simulink model "cam1"  (R2016b)
settings: Solver=ode3  StartTime=0.0  StopTime=1000.0  FixedStep=0.2  RelTol=1e-3  EnableMultiTasking=on
undefined symbols (not defined in the file or in its folder): Angular, Linear
libraries: robotlib x3, simulink x3, realtime_pacer_lib x2
settings Model: Creator=esther  LastModifiedBy=esther
settings DataIOCC: SaveFormat=Array
settings OptimizationCC: MaxStackSize=64
settings DebuggingCC: ParameterTunabilityLossMsg=error
settings HardwareCC: ProdBitPerPointer=32  ProdBitPerSizeT=32  ProdBitPerPtrDiffT=32  ProdLargestAtomicFloat=None  ProdIntDivRoundTo=Undefined  ProdEndianess=Unspecified  ProdWordSize=32  ProdHWDeviceType=Generic->Unspecified (assume 32-bit Generic)
settings RTWCC: SystemTargetFile=ert.tlc  HardwareBoard=Robot Operating System (ROS)  TLCOptions="-aInlineSetEventsForThisBaseRateFcn=TLC_FALSE -aSuppressMultiTaskScheduler=TLC_FALSE  -aRateBasedStepFcn=0"  TemplateMakefile=ert_default_tmf  Description=Embedded Coder  GenerateReport=on  RTWVerbose=off  Toolchain=Catkin  IncludeHyperlinkInReport=on  LaunchReport=on  TargetLang=C++  GenerateTraceInfo=on  GenerateTraceReport=on  GenerateTraceReportSl=on  GenerateTraceReportSf=on  GenerateTraceReportEml=on
settings CodeAppCC: ForceParamTrailComments=on  OperatorAnnotations=on  SimulinkDataObjDesc=on  SFDataObjDesc=on  MATLABFcnDesc=on  InsertBlockDesc=on  MATLABSourceComments=on
settings ERTTargetCC: MultiInstanceERTCode=on  CodeInterfacePackaging=C++ class  SupportContinuousTime=on  SupportVariableSizeSignals=on  RootIOFormat=Structure reference

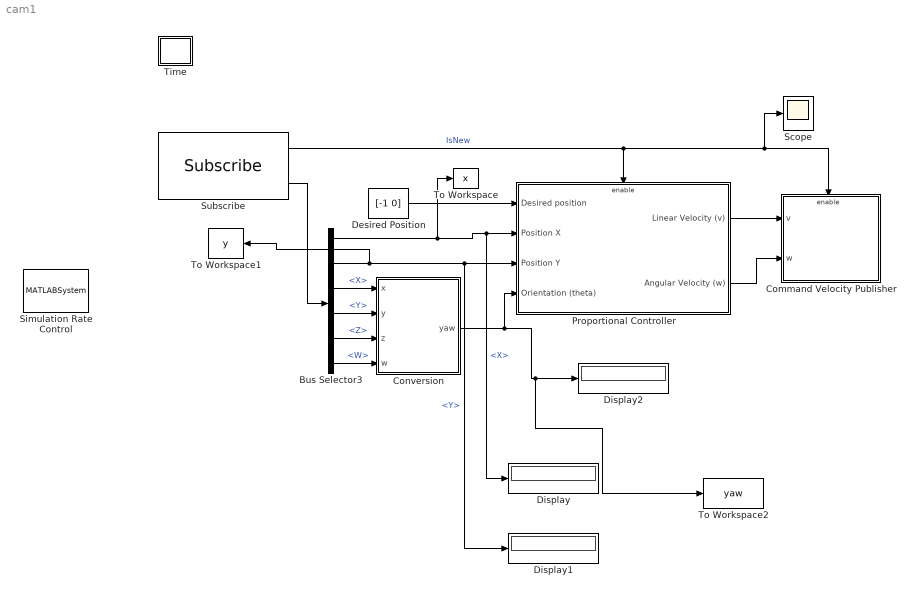
== system cam1 ==
  Bus Selector3 : BusSelector  OutputSignals=Pose.Pose.Position.X,Pose.Pose.Position.Y,Pose.Pose.Orientation.X,Pose.Pose.Orientation.Y,Pose.Pose.Orientation.Z,Pose.Pose.Orientation.W
  Command Velocity Publisher : Subsystem
  Conversion : MATLAB Function  TreatAsAtomicUnit=on
  Desired Position : Constant  Value=[-1 0]  SampleTime=-1
  Display : Display
  Display1 : Display
  Display2 : Display
  Proportional Controller : Subsystem
  Scope : Scope
  Simulation Rate Control : MATLABSystem  System=ExampleHelperSimulationRateControl  SampleTime=0.02
      mask Type: ExampleHelperSimulationRateControl
      mask Display: disp('Rate Control');
  Subscribe : robotlib/Subscribe  SourceLibraryInfo=This block requires Robotics System Toolbox  topicSource=Select from ROS network  topic=/robot_0/pose  messageType=nav_msgs/Odometry  sampleTime=-1  messageQueueLength=51
  Time : Subsystem
  To Workspace : ToWorkspace  VariableName=x  SampleTime=-1
  To Workspace1 : ToWorkspace  VariableName=y  SampleTime=-1
  To Workspace2 : ToWorkspace  VariableName=yaw  SampleTime=-1
  wires:
  Subscribe/2 -> Bus Selector3/1
  Desired Position/1 -> Proportional Controller/1(Desired position)
  Proportional Controller/1(Linear Velocity (v)) -> Command Velocity Publisher/1(v)
  Subscribe/1 -> Command Velocity Publisher/Enable, Scope/1, Proportional Controller/Enable  "IsNew"
  Bus Selector3/3 -> Conversion/1(x)  "<X>"
  Bus Selector3/4 -> Conversion/2(y)  "<Y>"
  Bus Selector3/5 -> Conversion/3(z)  "<Z>"
  Bus Selector3/6 -> Conversion/4(w)  "<W>"
  Conversion/1(yaw) -> Proportional Controller/4(Orientation (theta)), To Workspace2/1, Display2/1
  Bus Selector3/2 -> To Workspace1/1, Display1/1, Proportional Controller/3(Position Y)  "<Y>"
  Proportional Controller/2(Angular Velocity (w)) -> Command Velocity Publisher/2(w)
  Bus Selector3/1 -> To Workspace/1, Display/1, Proportional Controller/2(Position X)  "<X>"

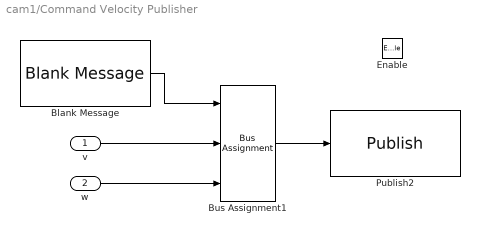
== system cam1/Command Velocity Publisher ==
  v : Inport
  w : Inport  Port=2
  Enable : EnablePort
  Blank Message : robotlib/Blank Message  SourceLibraryInfo=This block requires Robotics System Toolbox  messageType=geometry_msgs/Twist  SampleTime=inf
  Bus Assignment1 : BusAssignment  DialogController=Simulink.DDGSource_BusAssignment  AssignedSignals=Linear.X,Angular.Z
  Publish2 : robotlib/Publish  SourceLibraryInfo=This block requires Robotics System Toolbox  topicSource=Select from ROS network  topic=/robot_0/cmd_vel  messageType=geometry_msgs/Twist  messageQueueLength=105
  wires:
  Bus Assignment1/1 -> Publish2/1
  Blank Message/1 -> Bus Assignment1/1
  v/1 -> Bus Assignment1/2
  w/1 -> Bus Assignment1/3

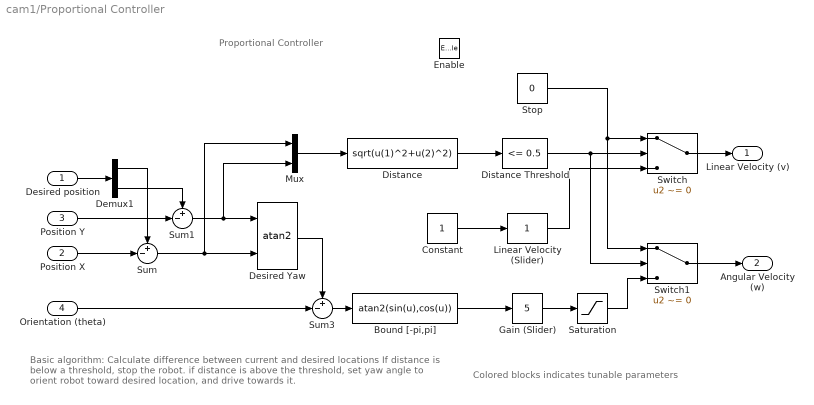
== system cam1/Proportional Controller ==
  note: Proportional Controller
  note: Basic algorithm:
      | Calculate difference between current and desired locations
      | If distance is below a threshold, stop the robot.
      | if distance is above the threshold, set yaw angle to orient robot toward desired location, and drive towards it.
  note: Colored blocks indicates tunable parameters
  Desired position : Inport
  Position X : Inport  Port=2
  Position Y : Inport  Port=3
  Orientation (theta) : Inport  Port=4
  Enable : EnablePort
  Bound [-pi,pi] : Fcn  Expr=atan2(sin(u),cos(u))
  Constant : Constant
  Demux1 : Demux  Outputs=2
  Desired Yaw : Trigonometry  Operator=atan2
  Distance : Fcn  Expr=sqrt(u(1)^2+u(2)^2)
  Distance Threshold : simulink/Logic and Bit Operations/Compare To Constant  relop=<=  const=0.5  OutDataTypeStr=boolean
  Gain (Slider) : simulink/Math Operations/Slider Gain  low=1  gain=5  high=10
  Linear Velocity (Slider) : simulink/Math Operations/Slider Gain  low=0  gain=1  high=2
  Mux : Mux  Inputs=2
  Saturation : Saturate
  Stop : Constant  Value=0
  Sum : Sum  Inputs=+-|
  Sum1 : Sum  Inputs=+-|
  Sum3 : Sum  Inputs=+-|
  Switch : Switch  Criteria=u2 ~= 0
  Switch1 : Switch  Criteria=u2 ~= 0
  Linear Velocity (v) : Outport
  Angular Velocity (w) : Outport  Port=2
  wires:
  Demux1/1 -> Sum/1
  Demux1/2 -> Sum1/1
  Sum1/1 -> Desired Yaw/1, Mux/2
  Constant/1 -> Linear Velocity (Slider)/1
  Desired position/1 -> Demux1/1
  Position Y/1 -> Sum1/2
  Position X/1 -> Sum/2
  Distance/1 -> Distance Threshold/1
  Mux/1 -> Distance/1
  Bound [-pi,pi]/1 -> Gain (Slider)/1
  Orientation (theta)/1 -> Sum3/2
  Desired Yaw/1 -> Sum3/1
  Sum/1 -> Desired Yaw/2, Mux/1
  Distance Threshold/1 -> Switch/2, Switch1/2
  Gain (Slider)/1 -> Saturation/1
  Saturation/1 -> Switch1/3
  Stop/1 -> Switch/1, Switch1/1
  Sum3/1 -> Bound [-pi,pi]/1
  Switch/1 -> Linear Velocity (v)/1
  Linear Velocity (Slider)/1 -> Switch/3
  Switch1/1 -> Angular Velocity (w)/1

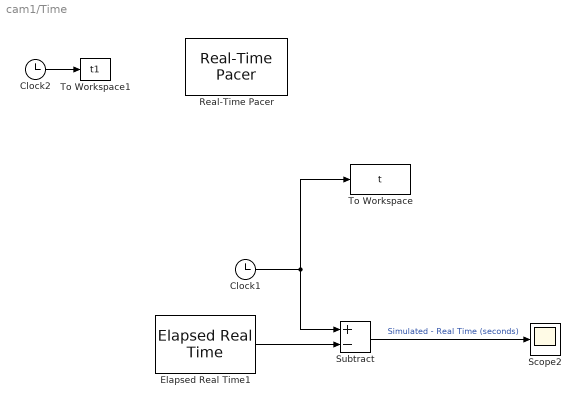
== system cam1/Time ==
  Clock1 : Clock
  Clock2 : Clock
  Elapsed Real Time1 : realtime_pacer_lib/Elapsed Real Time
  Real-Time Pacer : realtime_pacer_lib/Real-Time Pacer  simTimePerRealTime=1
  Scope2 : Scope
  Subtract : Sum  Inputs=+-
  To Workspace : ToWorkspace  VariableName=t  SaveFormat=Timeseries  SampleTime=-1
  To Workspace1 : ToWorkspace  VariableName=t1  SampleTime=-1
  wires:
  Elapsed Real Time1/1 -> Subtract/2
  Subtract/1 -> Scope2/1  "Simulated - Real Time (seconds)"
  Clock1/1 -> To Workspace/1, Subtract/1
  Clock2/1 -> To Workspace1/1

== matlab function cam1/Conversion ==
  data: yaw output; x input; y input; z input; w input
function yaw  = quat2eul(x,y,z,w)
%#codegen

% Convert the quaternion to a yaw angle (zyx euler angle)
eul = quat2eul([w,x,y,z]);
yaw = eul(1);

end
